simulink library "Lib_Turbo_PGenerator_TMATS"  (R2019b)
settings: Solver=ode45  StartTime=0.0  StopTime=10.0  RelTol=1e-3  EnableMultiTasking=on
Description:
  | Thomas Modules
settings Model: Creator=jwchapm2  LastModifiedBy=bhisma
settings DataIOCC: LimitDataPoints=on  SaveFormat=Array  ReturnWorkspaceOutputs=off
settings OptimizationCC: ExpressionDepthLimit=2147483647  LifeSpan=inf
settings DebuggingCC: UnderspecifiedInitializationDetection=Classic  MergeDetectMultiDrivingBlocksExec=none  SolverPrmCheckMsg=warning  StateNameClashWarn=warning  SFUnexpectedBacktrackingDiag=warning  SFNoUnconditionalDefaultTransitionDiag=warning  SFExecutionAtInitializationDiag=none  ArithmeticOperatorsInVariantConditions=warning
settings HardwareCC: ProdBitPerPointer=32  ProdBitPerSizeT=32  ProdBitPerPtrDiffT=32  ProdLargestAtomicFloat=None  ProdIntDivRoundTo=Undefined  ProdEndianess=Unspecified  ProdWordSize=32  ProdHWDeviceType=32-bit Generic
settings ModelReferenceCC: PropagateSignalLabelsOutOfModel=off
settings SFSimCC: SimUseLocalCustomCode=off  CustomCodeUndefinedFunction=UseInterfaceOnly
settings RTWCC: RTWUseLocalCustomCode=off
settings CodeAppCC: StateflowObjectComments=on
settings GRTTargetCC: TargetLangStandard=C89/C90 (ANSI)  GeneratePreprocessorConditionals=Disable all
settings ConfigComp: CovMetricSettings=dw  CovHtmlReporting=on  CovSaveCumulativeToWorkspaceVar=on  CovSaveSingleToWorkspaceVar=on  CovExternalEMLEnable=off

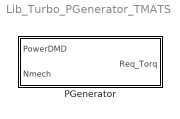
== system Lib_Turbo_PGenerator_TMATS ==
  PGenerator : Subsystem  mask(T-MATS: Power Generation Library Block){Eff_M=.995}
      mask prompts: Eff_M "Eff_M - Efficiency"
      mask help: This block converts a power demand with rotational speed into a torque and can be used to simulate a power generator.
      mask Help: web(which('Turbo_TMATS_PGen.html'),'-helpbrowser')

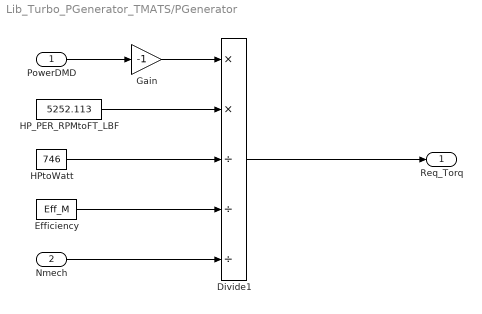
== system Lib_Turbo_PGenerator_TMATS/PGenerator ==
  PowerDMD : Inport
  Nmech : Inport  Port=2
  Divide1 : Product  Inputs=**///
  Efficiency : Constant  Value=Eff_M
  Gain : Gain  Gain=-1
  HP_PER_RPMtoFT_LBF : Constant  Value=5252.113
  HPtoWatt : Constant  Value=746
  Req_Torq : Outport
  wires:
  PowerDMD/1 -> Gain/1
  Divide1/1 -> Req_Torq/1
  Nmech/1 -> Divide1/5
  Gain/1 -> Divide1/1
  HPtoWatt/1 -> Divide1/3
  HP_PER_RPMtoFT_LBF/1 -> Divide1/2
  Efficiency/1 -> Divide1/4
